simulink model "ALL_JP360_DBW_V6_5_1103"  (R2022a)
settings: Solver=FixedStepAuto  StartTime=0.0  StopTime=inf  FixedStep=0.01  RelTol=1e-3  EnableMultiTasking=on
model workspace (MAT data in the model file):
  g = 9.8
undefined symbols (not defined in the file or in its folder): canChannel, delta_v_p, IPM_Line_C0, IPM_Line_C1, IPM_Line_C2, IPM_Line_C3, M, M_p, MRR_ObjDistX, MRR_ObjDistY, MRR_ObjFusionCamID, MRR_ObjFusionSig, MRR_ObjID, MRR_ObjRelVelX, MRR_ObjRelVelY, MRR_ObjType, MRR_ObjUpdFlg, none, obj_vaild, untracktime, V, videoinput
libraries: canfdmsglib x230, canfdlib x76, slpidlib x24, simulink x18, dspstat3 x14, ctrlSharedLib x1, simulink_extras x1, imaqlib x1, realtime_pacer_lib x1, dspvision x1, visionsinks x1
(part 34 of 55)

== system ALL_JP360_DBW_V6_5_1103/MsgFromCAN/SRR_ADCU_MsgFromCAN/SRR_ADCU_RRR_Freespace_0x1EC ==
  SRR_ADCU_RRR_Freespace_0x1ECFromInData : Inport  OutDataTypeStr=Bus:CAN_FD_MESSAGE_BUS
  Bus Creator : BusCreator  Inputs=104  OutDataTypeStr=Bus:SRR_ADCU_RRR_Freespace_0x1EC  NonVirtualBus=on
  CAN FD Unpack : canfdmsglib/CAN FD Unpack  CANdbFile=V363 SRR Private CAN-V1.3.dbc  MsgList=(none)  MsgName=RRR_Freespace_0x1EC  ProtocolMode=CAN FD  MsgIDType=Standard (11-bit identifier)  MsgIdentifier=492  MsgLength=64  SignalInfo={'RRR_CRCCheck_FSP_MSG2','504','16','BE','unsigned','Standard','0','1','0','0','65535';'RRR_FreespaceSectorConfidence35','12','2','BE','unsigned','Standard','0','1','0','0','3';'RRR_FreespaceSectorConfidence36','30','2','BE','unsigned','Standard','0','1','0','0','3';'RRR_FreespaceSectorConfidence37','32','2','BE','unsigned','Standard','0','1','0','0','3';'RRR_FreespaceSectorConfidence38','50','2','BE','unsigned','Standard','0','1','0','0','3';'RRR_FreespaceSectorConfidence39','68','2','BE','unsigned','Standard','0','1','0','0','3';'RRR_FreespaceSectorConfidence40','86','2','BE','unsigned','Standard','0','1','0','0','3';'RRR_FreespaceSectorConfidence41','88','2','BE','unsigned','Standard','0','1','0','0','3';'RRR_FreespaceSectorConfidence42','106','2','BE','unsigned','Standard','0','1','0','0','3';'RRR_FreespaceSectorConfidence43','124','2','BE','unsigned','Standard','0','1','0','0','3';'RRR_FreespaceSectorConfidence44','142','2','BE','unsigned','Standard','0','1','0','0','3';'RRR_FreespaceSectorConfidence45','144','2','BE','unsigned','Standard','0','1','0','0','3';'RRR_FreespaceSectorConfidence46','162','2','BE','unsigned','Standard','0','1','0','0','3';'RRR_FreespaceSectorConfidence47','180','2','BE','unsigned','Standard','0','1','0','0','3';'RRR_FreespaceSectorConfidence48','198','2','BE','unsigned','Standard','0','1','0','0','3';'RRR_FreespaceSectorConfidence49','200','2','BE','unsigned','Standard','0','1','0','0','3';'RRR_FreespaceSectorConfidence50','218','2','BE','unsigned','Standard','0','1','0','0','3';'RRR_FreespaceSectorConfidence51','236','2','BE','unsigned','Standard','0','1','0','0','3';'RRR_FreespaceSectorConfidence52','254','2','BE','unsigned','Standard','0','1','0','0','3';'RRR_FreespaceSectorConfidence53','256','2','BE','unsigned','Standard','0','1','0','0','3';'RRR_FreespaceSectorConfidence54','274','2','BE','unsigned','Standard','0','1','0','0','3';'RRR_FreespaceSectorConfidence55','292','2','BE','unsigned','Standard','0','1','0','0','3';'RRR_FreespaceSectorConfidence56','310','2','BE','unsigned','Standard','0','1','0','0','3';'RRR_FreespaceSectorConfidence57','312','2','BE','unsigned','Standard','0','1','0','0','3';'RRR_FreespaceSectorConfidence58','330','2','BE','unsigned','Standard','0','1','0','0','3';'RRR_FreespaceSectorConfidence59','348','2','BE','unsigned','Standard','0','1','0','0','3';'RRR_FreespaceSectorConfidence60','366','2','BE','unsigned','Standard','0','1','0','0','3';'RRR_FreespaceSectorConfidence61','368','2','BE','unsigned','Standard','0','1','0','0','3';'RRR_FreespaceSectorConfidence62','386','2','BE','unsigned','Standard','0','1','0','0','3';'RRR_FreespaceSectorConfidence63','404','2','BE','unsigned','Standard','0','1','0','0','3';'RRR_FreespaceSectorConfidence64','422','2','BE','unsigned','Standard','0','1','0','0','3';'RRR_FreespaceSectorConfidence65','424','2','BE','unsigned','Standard','0','1','0','0','3';'RRR_FreespaceSectorConfidence66','442','2','BE','unsigned','Standard','0','1','0','0','3';'RRR_FreespaceSectorConfidence67','460','2','BE','unsigned','Standard','0','1','0','0','3';'RRR_FreespaceSectorConfidence68','478','2','BE','unsigned','Standard','0','1','0','0','3';'RRR_FreespaceSectorDistance35','14','10','BE','unsigned','Standard','0','0.1','0','0','100';'RRR_FreespaceSectorDistance36','16','10','BE','unsigned','Standard','0','0.1','0','0','100';'RRR_FreespaceSectorDistance37','34','10','BE','unsigned','Standard','0','0.1','0','0','100';'RRR_FreespaceSectorDistance38','52','10','BE','unsigned','Standard','0','0.1','0','0','100';'RRR_FreespaceSectorDistance39','70','10','BE','unsigned','Standard','0','0.1','0','0','100';'RRR_FreespaceSectorDistance40','72','10','BE','unsigned','Standard','0','0.1','0','0','100';'RRR_FreespaceSectorDistance41','90','10','BE','unsigned','Standard','0','0.1','0','0','100';'RRR_FreespaceSectorDistance42','108','10','BE','unsigned','Standard','0','0.1','0','0','100';'RRR_FreespaceSectorDistance43','126','10','BE','unsigned','Standard','0','0.1','0','0','100';'RRR_FreespaceSectorDistance44','128','10','BE','unsigned','Standard','0','0.1','0','0','100';'RRR_FreespaceSectorDistance45','146','10','BE','unsigned','Standard','0','0.1','0','0','100';'RRR_FreespaceSectorDistance46','164','10','BE','unsigned','Standard','0','0.1','0','0','100';'RRR_FreespaceSectorDistance47','182','10','BE','unsigned','Standard','0','0.1','0','0','100';'RRR_FreespaceSectorDistance48','184','10','BE','unsigned','Standard','0','0.1','0','0','100';'RRR_FreespaceSectorDistance49','202','10','BE','unsigned','Standard','0','0.1','0','0','100';'RRR_FreespaceSectorDistance50','220','10','BE','unsigned','Standard','0','0.1','0','0','100';'RRR_FreespaceSectorDistance51','238','10','BE','unsigned','Standard','0','0.1','0','0','100';'RRR_FreespaceSectorDistance52','240','10','BE','unsigned','Standard','0','0.1','0','0','100';'RRR_FreespaceSectorDistance53','258','10','BE','unsigned','Standard','0','0.1','0','0','100';'RRR_FreespaceSectorDistance54','276','10','BE','unsigned','Standard','0','0.1','0','0','100';'RRR_FreespaceSectorDistance55','294','10','BE','unsigned','Standard','0','0.1','0','0','100';'RRR_FreespaceSectorDistance56','296','10','BE','unsigned','Standard','0','0.1','0','0','100';'RRR_FreespaceSectorDistance57','314','10','BE','unsigned','Standard','0','0.1','0','0','100';'RRR_FreespaceSectorDistance58','332','10','BE','unsigned','Standard','0','0.1','0','0','100';'RRR_FreespaceSectorDistance59','350','10','BE','unsigned','Standard','0','0.1','0','0','100';'RRR_FreespaceSectorDistance60','352','10','BE','unsigned','Standard','0','0.1','0','0','100';'RRR_FreespaceSectorDistance61','370','10','BE','unsigned','Standard','0','0.1','0','0','100';'RRR_FreespaceSectorDistance62','388','10','BE','unsigned','Standard','0','0.1','0','0','100';'RRR_FreespaceSectorDistance63','406','10','BE','unsigned','Standard','0','0.1','0','0','100';'RRR_FreespaceSectorDistance64','408','10','BE','unsigned','Standard','0','0.1','0','0','100';'RRR_FreespaceSectorDistance65','426','10','BE','unsigned','Standard','0','0.1','0','0','100';'RRR_FreespaceSectorDistance66','444','10','BE','unsigned','Standard','0','0.1','0','0','100';'RRR_FreespaceSectorDistance67','462','10','BE','unsigned','Standard','0','0.1','0','0','100';'RRR_FreespaceSectorDistance68','464','10','BE','unsigned','Standard','0','0.1','0','0','100';'RRR_FreespaceSectorKinestate35','10','2','BE','unsigned','Standard','0','1','0','0','3';'RRR_FreespaceSectorKinestate36','28','2','BE','unsigned','Standard','0','1','0','0','3';'RRR_FreespaceSectorKinestate37','46','2','BE','unsigned','Standard','0','1','0','0','3';'RRR_FreespaceSectorKinestate38','48','2','BE','unsigned','Standard','0','1','0','0','3';'RRR_FreespaceSectorKinestate39','66','2','BE','unsigned','Standard','0','1','0','0','3';'RRR_FreespaceSectorKinestate40','84','2','BE','unsigned','Standard','0','1','0','0','3';'RRR_FreespaceSectorKinestate41','102','2','BE','unsigned','Standard','0','1','0','0','3';'RRR_FreespaceSectorKinestate42','104','2','BE','unsigned','Standard','0','1','0','0','3';'RRR_FreespaceSectorKinestate43','122','2','BE','unsigned','Standard','0','1','0','0','3';'RRR_FreespaceSectorKinestate44','140','2','BE','unsigned','Standard','0','1','0','0','3';'RRR_FreespaceSectorKinestate45','158','2','BE','unsigned','Standard','0','1','0','0','3';'RRR_FreespaceSectorKinestate46','160','2','BE','unsigned','Standard','0','1','0','0','3';'RRR_FreespaceSectorKinestate47','178','2','BE','unsigned','Standard','0','1','0','0','3';'RRR_FreespaceSectorKinestate48','196','2','BE','unsigned','Standard','0','1','0','0','3';'RRR_FreespaceSectorKinestate49','214','2','BE','unsigned','Standard','0','1','0','0','3';'RRR_FreespaceSectorKinestate50','216','2','BE','unsigned','Standard','0','1','0','0','3';'RRR_FreespaceSectorKinestate51','234','2','BE','unsigned','Standard','0','1','0','0','3';'RRR_FreespaceSectorKinestate52','252','2','BE','unsigned','Standard','0','1','0','0','3';'RRR_FreespaceSectorKinestate53','270','2','BE','unsigned','Standard','0','1','0','0','3';'RRR_FreespaceSectorKinestate54','272','2','BE','unsigned','Standard','0','1','0','0','3';'RRR_FreespaceSectorKinestate55','290','2','BE','unsigned','Standard','0','1','0','0','3';'RRR_FreespaceSectorKinestate56','308','2','BE','unsigned','Standard','0','1','0','0','3';'RRR_FreespaceSectorKinestate57','326','2','BE','unsigned','Standard','0','1','0','0','3';'RRR_FreespaceSectorKinestate58','328','2','BE','unsigned','Standard','0','1','0','0','3';'RRR_FreespaceSectorKinestate59','346','2','BE','unsigned','Standard','0','1','0','0','3';'RRR_FreespaceSectorKinestate60','364','2','BE','unsigned','Standard','0','1','0','0','3';'RRR_FreespaceSectorKinestate61','382','2','BE','unsigned','Standard','0','1','0','0','3';'RRR_FreespaceSectorKinestate62','384','2','BE','unsigned','Standard','0','1','0','0','3';'RRR_FreespaceSectorKinestate63','402','2','BE','unsigned','Standard','0','1','0','0','3';'RRR_FreespaceSectorKinestate64','420','2','BE','unsigned','Standard','0','1','0','0','3';'RRR_FreespaceSectorKinestate65','438','2','BE','unsigned','Standard','0','1','0','0','3';'RRR_FreespaceSectorKinestate66','440','2','BE','unsigned','Standard','0','1','0','0','3';'RRR_FreespaceSectorKinestate67','458','2','BE','unsigned','Standard','0','1','0','0','3';'RRR_FreespaceSectorKinestate68','476','2','BE','unsigned','Standard','0','1','0','0','3';'RRR_RollingCounter_FSP_MSG2','488','4','BE','unsigned','Standard','0','1','0','0','15'}  IDPort=off  TimestampPort=off  ErrorPort=off  RemotePort=off  LengthPort=off  StatusPort=off  BRSPort=off  ESIPort=off  DLCPort=off  ApplyMinMax=off
      settings: SourceProductBaseCode=ME,XP,VN  DataFormat=CANdb specified signals
  Data Type Conversion1 : DataTypeConversion  OutDataTypeStr=uint16  SaturateOnIntegerOverflow=off  RndMeth=Floor
  Data Type Conversion{2..35,70..104} (69 alike) : DataTypeConversion  OutDataTypeStr=int8  SaturateOnIntegerOverflow=off  RndMeth=Floor
  Data Type Conversion{36..69} (34 alike) : DataTypeConversion  OutDataTypeStr=single  SaturateOnIntegerOverflow=off  RndMeth=Floor
  SRR_ADCU_RRR_Freespace_0x1ECFromOutData : Outport  OutDataTypeStr=Bus:SRR_ADCU_RRR_Freespace_0x1EC
  wires:
  CAN FD Unpack/1 -> Data Type Conversion1/1
  CAN FD Unpack/2 -> Data Type Conversion2/1
  CAN FD Unpack/3 -> Data Type Conversion3/1
  CAN FD Unpack/4 -> Data Type Conversion4/1
  CAN FD Unpack/5 -> Data Type Conversion5/1
  CAN FD Unpack/6 -> Data Type Conversion6/1
  CAN FD Unpack/7 -> Data Type Conversion7/1
  CAN FD Unpack/8 -> Data Type Conversion8/1
  CAN FD Unpack/9 -> Data Type Conversion9/1
  CAN FD Unpack/10 -> Data Type Conversion10/1
  CAN FD Unpack/11 -> Data Type Conversion11/1
  CAN FD Unpack/12 -> Data Type Conversion12/1
  CAN FD Unpack/13 -> Data Type Conversion13/1
  CAN FD Unpack/14 -> Data Type Conversion14/1
  CAN FD Unpack/15 -> Data Type Conversion15/1
  CAN FD Unpack/16 -> Data Type Conversion16/1
  CAN FD Unpack/17 -> Data Type Conversion17/1
  CAN FD Unpack/18 -> Data Type Conversion18/1
  CAN FD Unpack/19 -> Data Type Conversion19/1
  CAN FD Unpack/20 -> Data Type Conversion20/1
  CAN FD Unpack/21 -> Data Type Conversion21/1
  CAN FD Unpack/22 -> Data Type Conversion22/1
  CAN FD Unpack/23 -> Data Type Conversion23/1
  CAN FD Unpack/24 -> Data Type Conversion24/1
  CAN FD Unpack/25 -> Data Type Conversion25/1
  CAN FD Unpack/26 -> Data Type Conversion26/1
  CAN FD Unpack/27 -> Data Type Conversion27/1
  CAN FD Unpack/28 -> Data Type Conversion28/1
  CAN FD Unpack/29 -> Data Type Conversion29/1
  CAN FD Unpack/30 -> Data Type Conversion30/1
  CAN FD Unpack/31 -> Data Type Conversion31/1
  CAN FD Unpack/32 -> Data Type Conversion32/1
  CAN FD Unpack/33 -> Data Type Conversion33/1
  CAN FD Unpack/34 -> Data Type Conversion34/1
  CAN FD Unpack/35 -> Data Type Conversion35/1
  CAN FD Unpack/36 -> Data Type Conversion36/1
  CAN FD Unpack/37 -> Data Type Conversion37/1
  CAN FD Unpack/38 -> Data Type Conversion38/1
  CAN FD Unpack/39 -> Data Type Conversion39/1
  CAN FD Unpack/40 -> Data Type Conversion40/1
  CAN FD Unpack/41 -> Data Type Conversion41/1
  CAN FD Unpack/42 -> Data Type Conversion42/1
  CAN FD Unpack/43 -> Data Type Conversion43/1
  CAN FD Unpack/44 -> Data Type Conversion44/1
  CAN FD Unpack/45 -> Data Type Conversion45/1
  CAN FD Unpack/46 -> Data Type Conversion46/1
  CAN FD Unpack/47 -> Data Type Conversion47/1
  CAN FD Unpack/48 -> Data Type Conversion48/1
  CAN FD Unpack/49 -> Data Type Conversion49/1
  CAN FD Unpack/50 -> Data Type Conversion50/1
  CAN FD Unpack/51 -> Data Type Conversion51/1
  CAN FD Unpack/52 -> Data Type Conversion52/1
  CAN FD Unpack/53 -> Data Type Conversion53/1
  CAN FD Unpack/54 -> Data Type Conversion54/1
  CAN FD Unpack/55 -> Data Type Conversion55/1
  CAN FD Unpack/56 -> Data Type Conversion56/1
  CAN FD Unpack/57 -> Data Type Conversion57/1
  CAN FD Unpack/58 -> Data Type Conversion58/1
  CAN FD Unpack/59 -> Data Type Conversion59/1
  CAN FD Unpack/60 -> Data Type Conversion60/1
  CAN FD Unpack/61 -> Data Type Conversion61/1
  CAN FD Unpack/62 -> Data Type Conversion62/1
  CAN FD Unpack/63 -> Data Type Conversion63/1
  CAN FD Unpack/64 -> Data Type Conversion64/1
  CAN FD Unpack/65 -> Data Type Conversion65/1
  CAN FD Unpack/66 -> Data Type Conversion66/1
  CAN FD Unpack/67 -> Data Type Conversion67/1
  CAN FD Unpack/68 -> Data Type Conversion68/1
  CAN FD Unpack/69 -> Data Type Conversion69/1
  CAN FD Unpack/70 -> Data Type Conversion70/1
  CAN FD Unpack/71 -> Data Type Conversion71/1
  CAN FD Unpack/72 -> Data Type Conversion72/1
  CAN FD Unpack/73 -> Data Type Conversion73/1
  CAN FD Unpack/74 -> Data Type Conversion74/1
  CAN FD Unpack/75 -> Data Type Conversion75/1
  CAN FD Unpack/76 -> Data Type Conversion76/1
  CAN FD Unpack/77 -> Data Type Conversion77/1
  CAN FD Unpack/78 -> Data Type Conversion78/1
  CAN FD Unpack/79 -> Data Type Conversion79/1
  CAN FD Unpack/80 -> Data Type Conversion80/1
  CAN FD Unpack/81 -> Data Type Conversion81/1
  CAN FD Unpack/82 -> Data Type Conversion82/1
  CAN FD Unpack/83 -> Data Type Conversion83/1
  CAN FD Unpack/84 -> Data Type Conversion84/1
  CAN FD Unpack/85 -> Data Type Conversion85/1
  CAN FD Unpack/86 -> Data Type Conversion86/1
  CAN FD Unpack/87 -> Data Type Conversion87/1
  CAN FD Unpack/88 -> Data Type Conversion88/1
  CAN FD Unpack/89 -> Data Type Conversion89/1
  CAN FD Unpack/90 -> Data Type Conversion90/1
  CAN FD Unpack/91 -> Data Type Conversion91/1
  CAN FD Unpack/92 -> Data Type Conversion92/1
  CAN FD Unpack/93 -> Data Type Conversion93/1
  CAN FD Unpack/94 -> Data Type Conversion94/1
  CAN FD Unpack/95 -> Data Type Conversion95/1
  CAN FD Unpack/96 -> Data Type Conversion96/1
  CAN FD Unpack/97 -> Data Type Conversion97/1
  CAN FD Unpack/98 -> Data Type Conversion98/1
  CAN FD Unpack/99 -> Data Type Conversion99/1
  CAN FD Unpack/100 -> Data Type Conversion100/1
  CAN FD Unpack/101 -> Data Type Conversion101/1
  CAN FD Unpack/102 -> Data Type Conversion102/1
  CAN FD Unpack/103 -> Data Type Conversion103/1
  CAN FD Unpack/104 -> Data Type Conversion104/1
  Data Type Conversion1/1 -> Bus Creator/1  "RRR_CRCCheck_FSP_MSG2"
  Data Type Conversion2/1 -> Bus Creator/2  "RRR_FreespaceSectorConfidence35"
  Data Type Conversion3/1 -> Bus Creator/3  "RRR_FreespaceSectorConfidence36"
  Data Type Conversion4/1 -> Bus Creator/4  "RRR_FreespaceSectorConfidence37"
  Data Type Conversion5/1 -> Bus Creator/5  "RRR_FreespaceSectorConfidence38"
  Data Type Conversion6/1 -> Bus Creator/6  "RRR_FreespaceSectorConfidence39"
  Data Type Conversion7/1 -> Bus Creator/7  "RRR_FreespaceSectorConfidence40"
  Data Type Conversion8/1 -> Bus Creator/8  "RRR_FreespaceSectorConfidence41"
  Data Type Conversion9/1 -> Bus Creator/9  "RRR_FreespaceSectorConfidence42"
  Data Type Conversion10/1 -> Bus Creator/10  "RRR_FreespaceSectorConfidence43"
  Data Type Conversion11/1 -> Bus Creator/11  "RRR_FreespaceSectorConfidence44"
  Data Type Conversion12/1 -> Bus Creator/12  "RRR_FreespaceSectorConfidence45"
  Data Type Conversion13/1 -> Bus Creator/13  "RRR_FreespaceSectorConfidence46"
  Data Type Conversion14/1 -> Bus Creator/14  "RRR_FreespaceSectorConfidence47"
  Data Type Conversion15/1 -> Bus Creator/15  "RRR_FreespaceSectorConfidence48"
  Data Type Conversion16/1 -> Bus Creator/16  "RRR_FreespaceSectorConfidence49"
  Data Type Conversion17/1 -> Bus Creator/17  "RRR_FreespaceSectorConfidence50"
  Data Type Conversion18/1 -> Bus Creator/18  "RRR_FreespaceSectorConfidence51"
  Data Type Conversion19/1 -> Bus Creator/19  "RRR_FreespaceSectorConfidence52"
  Data Type Conversion20/1 -> Bus Creator/20  "RRR_FreespaceSectorConfidence53"
  Data Type Conversion21/1 -> Bus Creator/21  "RRR_FreespaceSectorConfidence54"
  Data Type Conversion22/1 -> Bus Creator/22  "RRR_FreespaceSectorConfidence55"
  Data Type Conversion23/1 -> Bus Creator/23  "RRR_FreespaceSectorConfidence56"
  Data Type Conversion24/1 -> Bus Creator/24  "RRR_FreespaceSectorConfidence57"
  Data Type Conversion25/1 -> Bus Creator/25  "RRR_FreespaceSectorConfidence58"
  Data Type Conversion26/1 -> Bus Creator/26  "RRR_FreespaceSectorConfidence59"
  Data Type Conversion27/1 -> Bus Creator/27  "RRR_FreespaceSectorConfidence60"
  Data Type Conversion28/1 -> Bus Creator/28  "RRR_FreespaceSectorConfidence61"
  Data Type Conversion29/1 -> Bus Creator/29  "RRR_FreespaceSectorConfidence62"
  Data Type Conversion30/1 -> Bus Creator/30  "RRR_FreespaceSectorConfidence63"
  Data Type Conversion31/1 -> Bus Creator/31  "RRR_FreespaceSectorConfidence64"
  Data Type Conversion32/1 -> Bus Creator/32  "RRR_FreespaceSectorConfidence65"
  Data Type Conversion33/1 -> Bus Creator/33  "RRR_FreespaceSectorConfidence66"
  Data Type Conversion34/1 -> Bus Creator/34  "RRR_FreespaceSectorConfidence67"
  Data Type Conversion35/1 -> Bus Creator/35  "RRR_FreespaceSectorConfidence68"
  Data Type Conversion36/1 -> Bus Creator/36  "RRR_FreespaceSectorDistance35"
  Data Type Conversion37/1 -> Bus Creator/37  "RRR_FreespaceSectorDistance36"
  Data Type Conversion38/1 -> Bus Creator/38  "RRR_FreespaceSectorDistance37"
  Data Type Conversion39/1 -> Bus Creator/39  "RRR_FreespaceSectorDistance38"
  Data Type Conversion40/1 -> Bus Creator/40  "RRR_FreespaceSectorDistance39"
  Data Type Conversion41/1 -> Bus Creator/41  "RRR_FreespaceSectorDistance40"
  Data Type Conversion42/1 -> Bus Creator/42  "RRR_FreespaceSectorDistance41"
  Data Type Conversion43/1 -> Bus Creator/43  "RRR_FreespaceSectorDistance42"
  Data Type Conversion44/1 -> Bus Creator/44  "RRR_FreespaceSectorDistance43"
  Data Type Conversion45/1 -> Bus Creator/45  "RRR_FreespaceSectorDistance44"
  Data Type Conversion46/1 -> Bus Creator/46  "RRR_FreespaceSectorDistance45"
  Data Type Conversion47/1 -> Bus Creator/47  "RRR_FreespaceSectorDistance46"
  Data Type Conversion48/1 -> Bus Creator/48  "RRR_FreespaceSectorDistance47"
  Data Type Conversion49/1 -> Bus Creator/49  "RRR_FreespaceSectorDistance48"
  Data Type Conversion50/1 -> Bus Creator/50  "RRR_FreespaceSectorDistance49"
  Data Type Conversion51/1 -> Bus Creator/51  "RRR_FreespaceSectorDistance50"
  Data Type Conversion52/1 -> Bus Creator/52  "RRR_FreespaceSectorDistance51"
  Data Type Conversion53/1 -> Bus Creator/53  "RRR_FreespaceSectorDistance52"
  Data Type Conversion54/1 -> Bus Creator/54  "RRR_FreespaceSectorDistance53"
  Data Type Conversion55/1 -> Bus Creator/55  "RRR_FreespaceSectorDistance54"
  Data Type Conversion56/1 -> Bus Creator/56  "RRR_FreespaceSectorDistance55"
  Data Type Conversion57/1 -> Bus Creator/57  "RRR_FreespaceSectorDistance56"
  Data Type Conversion58/1 -> Bus Creator/58  "RRR_FreespaceSectorDistance57"
  Data Type Conversion59/1 -> Bus Creator/59  "RRR_FreespaceSectorDistance58"
  Data Type Conversion60/1 -> Bus Creator/60  "RRR_FreespaceSectorDistance59"
  Data Type Conversion61/1 -> Bus Creator/61  "RRR_FreespaceSectorDistance60"
  Data Type Conversion62/1 -> Bus Creator/62  "RRR_FreespaceSectorDistance61"
  Data Type Conversion63/1 -> Bus Creator/63  "RRR_FreespaceSectorDistance62"
  Data Type Conversion64/1 -> Bus Creator/64  "RRR_FreespaceSectorDistance63"
  Data Type Conversion65/1 -> Bus Creator/65  "RRR_FreespaceSectorDistance64"
  Data Type Conversion66/1 -> Bus Creator/66  "RRR_FreespaceSectorDistance65"
  Data Type Conversion67/1 -> Bus Creator/67  "RRR_FreespaceSectorDistance66"
  Data Type Conversion68/1 -> Bus Creator/68  "RRR_FreespaceSectorDistance67"
  Data Type Conversion69/1 -> Bus Creator/69  "RRR_FreespaceSectorDistance68"
  Data Type Conversion70/1 -> Bus Creator/70  "RRR_FreespaceSectorKinestate35"
  Data Type Conversion71/1 -> Bus Creator/71  "RRR_FreespaceSectorKinestate36"
  Data Type Conversion72/1 -> Bus Creator/72  "RRR_FreespaceSectorKinestate37"
  Data Type Conversion73/1 -> Bus Creator/73  "RRR_FreespaceSectorKinestate38"
  Data Type Conversion74/1 -> Bus Creator/74  "RRR_FreespaceSectorKinestate39"
  Data Type Conversion75/1 -> Bus Creator/75  "RRR_FreespaceSectorKinestate40"
  Data Type Conversion76/1 -> Bus Creator/76  "RRR_FreespaceSectorKinestate41"
  Data Type Conversion77/1 -> Bus Creator/77  "RRR_FreespaceSectorKinestate42"
  Data Type Conversion78/1 -> Bus Creator/78  "RRR_FreespaceSectorKinestate43"
  Data Type Conversion79/1 -> Bus Creator/79  "RRR_FreespaceSectorKinestate44"
  Data Type Conversion80/1 -> Bus Creator/80  "RRR_FreespaceSectorKinestate45"
  Data Type Conversion81/1 -> Bus Creator/81  "RRR_FreespaceSectorKinestate46"
  Data Type Conversion82/1 -> Bus Creator/82  "RRR_FreespaceSectorKinestate47"
  Data Type Conversion83/1 -> Bus Creator/83  "RRR_FreespaceSectorKinestate48"
  Data Type Conversion84/1 -> Bus Creator/84  "RRR_FreespaceSectorKinestate49"
  Data Type Conversion85/1 -> Bus Creator/85  "RRR_FreespaceSectorKinestate50"
  Data Type Conversion86/1 -> Bus Creator/86  "RRR_FreespaceSectorKinestate51"
  Data Type Conversion87/1 -> Bus Creator/87  "RRR_FreespaceSectorKinestate52"
  Data Type Conversion88/1 -> Bus Creator/88  "RRR_FreespaceSectorKinestate53"
  Data Type Conversion89/1 -> Bus Creator/89  "RRR_FreespaceSectorKinestate54"
  Data Type Conversion90/1 -> Bus Creator/90  "RRR_FreespaceSectorKinestate55"
  Data Type Conversion91/1 -> Bus Creator/91  "RRR_FreespaceSectorKinestate56"
  Data Type Conversion92/1 -> Bus Creator/92  "RRR_FreespaceSectorKinestate57"
  Data Type Conversion93/1 -> Bus Creator/93  "RRR_FreespaceSectorKinestate58"
  Data Type Conversion94/1 -> Bus Creator/94  "RRR_FreespaceSectorKinestate59"
  Data Type Conversion95/1 -> Bus Creator/95  "RRR_FreespaceSectorKinestate60"
  Data Type Conversion96/1 -> Bus Creator/96  "RRR_FreespaceSectorKinestate61"
  Data Type Conversion97/1 -> Bus Creator/97  "RRR_FreespaceSectorKinestate62"
  Data Type Conversion98/1 -> Bus Creator/98  "RRR_FreespaceSectorKinestate63"
  Data Type Conversion99/1 -> Bus Creator/99  "RRR_FreespaceSectorKinestate64"
  Data Type Conversion100/1 -> Bus Creator/100  "RRR_FreespaceSectorKinestate65"
  Data Type Conversion101/1 -> Bus Creator/101  "RRR_FreespaceSectorKinestate66"
  Data Type Conversion102/1 -> Bus Creator/102  "RRR_FreespaceSectorKinestate67"
  Data Type Conversion103/1 -> Bus Creator/103  "RRR_FreespaceSectorKinestate68"
  Data Type Conversion104/1 -> Bus Creator/104  "RRR_RollingCounter_FSP_MSG2"
  Bus Creator/1 -> SRR_ADCU_RRR_Freespace_0x1ECFromOutData/1  "SRR_ADCU_RRR_Freespace_0x1ECFromOutData"
  SRR_ADCU_RRR_Freespace_0x1ECFromInData/1 -> CAN FD Unpack/1  "SRR_ADCU_RRR_Freespace_0x1ECFromInData"

== system ALL_JP360_DBW_V6_5_1103/MsgFromCAN/SRR_ADCU_MsgFromCAN/SRR_ADCU_RRR_Freespace_0x1ED ==
  SRR_ADCU_RRR_Freespace_0x1EDFromInData : Inport  OutDataTypeStr=Bus:CAN_FD_MESSAGE_BUS
  Bus Creator : BusCreator  Inputs=104  OutDataTypeStr=Bus:SRR_ADCU_RRR_Freespace_0x1ED  NonVirtualBus=on
  CAN FD Unpack : canfdmsglib/CAN FD Unpack  CANdbFile=V363 SRR Private CAN-V1.3.dbc  MsgList=(none)  MsgName=RRR_Freespace_0x1ED  ProtocolMode=CAN FD  MsgIDType=Standard (11-bit identifier)  MsgIdentifier=493  MsgLength=64  SignalInfo={'RRR_CRCCheck_FSP_MSG3','504','16','BE','unsigned','Standard','0','1','0','0','65535';'RRR_FreespaceSectorConfidence100','442','2','BE','unsigned','Standard','0','1','0','0','3';'RRR_FreespaceSectorConfidence101','460','2','BE','unsigned','Standard','0','1','0','0','3';'RRR_FreespaceSectorConfidence102','478','2','BE','unsigned','Standard','0','1','0','0','3';'RRR_FreespaceSectorConfidence69','12','2','BE','unsigned','Standard','0','1','0','0','3';'RRR_FreespaceSectorConfidence70','30','2','BE','unsigned','Standard','0','1','0','0','3';'RRR_FreespaceSectorConfidence71','32','2','BE','unsigned','Standard','0','1','0','0','3';'RRR_FreespaceSectorConfidence72','50','2','BE','unsigned','Standard','0','1','0','0','3';'RRR_FreespaceSectorConfidence73','68','2','BE','unsigned','Standard','0','1','0','0','3';'RRR_FreespaceSectorConfidence74','86','2','BE','unsigned','Standard','0','1','0','0','3';'RRR_FreespaceSectorConfidence75','88','2','BE','unsigned','Standard','0','1','0','0','3';'RRR_FreespaceSectorConfidence76','106','2','BE','unsigned','Standard','0','1','0','0','3';'RRR_FreespaceSectorConfidence77','124','2','BE','unsigned','Standard','0','1','0','0','3';'RRR_FreespaceSectorConfidence78','142','2','BE','unsigned','Standard','0','1','0','0','3';'RRR_FreespaceSectorConfidence79','144','2','BE','unsigned','Standard','0','1','0','0','3';'RRR_FreespaceSectorConfidence80','162','2','BE','unsigned','Standard','0','1','0','0','3';'RRR_FreespaceSectorConfidence81','180','2','BE','unsigned','Standard','0','1','0','0','3';'RRR_FreespaceSectorConfidence82','198','2','BE','unsigned','Standard','0','1','0','0','3';'RRR_FreespaceSectorConfidence83','200','2','BE','unsigned','Standard','0','1','0','0','3';'RRR_FreespaceSectorConfidence84','218','2','BE','unsigned','Standard','0','1','0','0','3';'RRR_FreespaceSectorConfidence85','236','2','BE','unsigned','Standard','0','1','0','0','3';'RRR_FreespaceSectorConfidence86','254','2','BE','unsigned','Standard','0','1','0','0','3';'RRR_FreespaceSectorConfidence87','256','2','BE','unsigned','Standard','0','1','0','0','3';'RRR_FreespaceSectorConfidence88','274','2','BE','unsigned','Standard','0','1','0','0','3';'RRR_FreespaceSectorConfidence89','292','2','BE','unsigned','Standard','0','1','0','0','3';'RRR_FreespaceSectorConfidence90','310','2','BE','unsigned','Standard','0','1','0','0','3';'RRR_FreespaceSectorConfidence91','312','2','BE','unsigned','Standard','0','1','0','0','3';'RRR_FreespaceSectorConfidence92','330','2','BE','unsigned','Standard','0','1','0','0','3';'RRR_FreespaceSectorConfidence93','348','2','BE','unsigned','Standard','0','1','0','0','3';'RRR_FreespaceSectorConfidence94','366','2','BE','unsigned','Standard','0','1','0','0','3';'RRR_FreespaceSectorConfidence95','368','2','BE','unsigned','Standard','0','1','0','0','3';'RRR_FreespaceSectorConfidence96','386','2','BE','unsigned','Standard','0','1','0','0','3';'RRR_FreespaceSectorConfidence97','404','2','BE','unsigned','Standard','0','1','0','0','3';'RRR_FreespaceSectorConfidence98','422','2','BE','unsigned','Standard','0','1','0','0','3';'RRR_FreespaceSectorConfidence99','424','2','BE','unsigned','Standard','0','1','0','0','3';'RRR_FreespaceSectorDistance100','444','10','BE','unsigned','Standard','0','0.1','0','0','100';'RRR_FreespaceSectorDistance101','462','10','BE','unsigned','Standard','0','0.1','0','0','100';'RRR_FreespaceSectorDistance102','464','10','BE','unsigned','Standard','0','0.1','0','0','100';'RRR_FreespaceSectorDistance69','14','10','BE','unsigned','Standard','0','0.1','0','0','100';'RRR_FreespaceSectorDistance70','16','10','BE','unsigned','Standard','0','0.1','0','0','100';'RRR_FreespaceSectorDistance71','34','10','BE','unsigned','Standard','0','0.1','0','0','100';'RRR_FreespaceSectorDistance72','52','10','BE','unsigned','Standard','0','0.1','0','0','100';'RRR_FreespaceSectorDistance73','70','10','BE','unsigned','Standard','0','0.1','0','0','100';'RRR_FreespaceSectorDistance74','72','10','BE','unsigned','Standard','0','0.1','0','0','100';'RRR_FreespaceSectorDistance75','90','10','BE','unsigned','Standard','0','0.1','0','0','100';'RRR_FreespaceSectorDistance76','108','10','BE','unsigned','Standard','0','0.1','0','0','100';'RRR_FreespaceSectorDistance77','126','10','BE','unsigned','Standard','0','0.1','0','0','100';'RRR_FreespaceSectorDistance78','128','10','BE','unsigned','Standard','0','0.1','0','0','100';'RRR_FreespaceSectorDistance79','146','10','BE','unsigned','Standard','0','0.1','0','0','100';'RRR_FreespaceSectorDistance80','164','10','BE','unsigned','Standard','0','0.1','0','0','100';'RRR_FreespaceSectorDistance81','182','10','BE','unsigned','Standard','0','0.1','0','0','100';'RRR_FreespaceSectorDistance82','184','10','BE','unsigned','Standard','0','0.1','0','0','100';'RRR_FreespaceSectorDistance83','202','10','BE','unsigned','Standard','0','0.1','0','0','100';'RRR_FreespaceSectorDistance84','220','10','BE','unsigned','Standard','0','0.1','0','0','100';'RRR_FreespaceSectorDistance85','238','10','BE','unsigned','Standard','0','0.1','0','0','100';'RRR_FreespaceSectorDistance86','240','10','BE','unsigned','Standard','0','0.1','0','0','100';'RRR_FreespaceSectorDistance87','258','10','BE','unsigned','Standard','0','0.1','0','0','100';'RRR_FreespaceSectorDistance88','276','10','BE','unsigned','Standard','0','0.1','0','0','100';'RRR_FreespaceSectorDistance89','294','10','BE','unsigned','Standard','0','0.1','0','0','100';'RRR_FreespaceSectorDistance90','296','10','BE','unsigned','Standard','0','0.1','0','0','100';'RRR_FreespaceSectorDistance91','314','10','BE','unsigned','Standard','0','0.1','0','0','100';'RRR_FreespaceSectorDistance92','332','10','BE','unsigned','Standard','0','0.1','0','0','100';'RRR_FreespaceSectorDistance93','350','10','BE','unsigned','Standard','0','0.1','0','0','100';'RRR_FreespaceSectorDistance94','352','10','BE','unsigned','Standard','0','0.1','0','0','100';'RRR_FreespaceSectorDistance95','370','10','BE','unsigned','Standard','0','0.1','0','0','100';'RRR_FreespaceSectorDistance96','388','10','BE','unsigned','Standard','0','0.1','0','0','100';'RRR_FreespaceSectorDistance97','406','10','BE','unsigned','Standard','0','0.1','0','0','100';'RRR_FreespaceSectorDistance98','408','10','BE','unsigned','Standard','0','0.1','0','0','100';'RRR_FreespaceSectorDistance99','426','10','BE','unsigned','Standard','0','0.1','0','0','100';'RRR_FreespaceSectorKinestate100','440','2','BE','unsigned','Standard','0','1','0','0','3';'RRR_FreespaceSectorKinestate101','458','2','BE','unsigned','Standard','0','1','0','0','3';'RRR_FreespaceSectorKinestate102','476','2','BE','unsigned','Standard','0','1','0','0','3';'RRR_FreespaceSectorKinestate69','10','2','BE','unsigned','Standard','0','1','0','0','3';'RRR_FreespaceSectorKinestate70','28','2','BE','unsigned','Standard','0','1','0','0','3';'RRR_FreespaceSectorKinestate71','46','2','BE','unsigned','Standard','0','1','0','0','3';'RRR_FreespaceSectorKinestate72','48','2','BE','unsigned','Standard','0','1','0','0','3';'RRR_FreespaceSectorKinestate73','66','2','BE','unsigned','Standard','0','1','0','0','3';'RRR_FreespaceSectorKinestate74','84','2','BE','unsigned','Standard','0','1','0','0','3';'RRR_FreespaceSectorKinestate75','102','2','BE','unsigned','Standard','0','1','0','0','3';'RRR_FreespaceSectorKinestate76','104','2','BE','unsigned','Standard','0','1','0','0','3';'RRR_FreespaceSectorKinestate77','122','2','BE','unsigned','Standard','0','1','0','0','3';'RRR_FreespaceSectorKinestate78','140','2','BE','unsigned','Standard','0','1','0','0','3';'RRR_FreespaceSectorKinestate79','158','2','BE','unsigned','Standard','0','1','0','0','3';'RRR_FreespaceSectorKinestate80','160','2','BE','unsigned','Standard','0','1','0','0','3';'RRR_FreespaceSectorKinestate81','178','2','BE','unsigned','Standard','0','1','0','0','3';'RRR_FreespaceSectorKinestate82','196','2','BE','unsigned','Standard','0','1','0','0','3';'RRR_FreespaceSectorKinestate83','214','2','BE','unsigned','Standard','0','1','0','0','3';'RRR_FreespaceSectorKinestate84','216','2','BE','unsigned','Standard','0','1','0','0','3';'RRR_FreespaceSectorKinestate85','234','2','BE','unsigned','Standard','0','1','0','0','3';'RRR_FreespaceSectorKinestate86','252','2','BE','unsigned','Standard','0','1','0','0','3';'RRR_FreespaceSectorKinestate87','270','2','BE','unsigned','Standard','0','1','0','0','3';'RRR_FreespaceSectorKinestate88','272','2','BE','unsigned','Standard','0','1','0','0','3';'RRR_FreespaceSectorKinestate89','290','2','BE','unsigned','Standard','0','1','0','0','3';'RRR_FreespaceSectorKinestate90','308','2','BE','unsigned','Standard','0','1','0','0','3';'RRR_FreespaceSectorKinestate91','326','2','BE','unsigned','Standard','0','1','0','0','3';'RRR_FreespaceSectorKinestate92','328','2','BE','unsigned','Standard','0','1','0','0','3';'RRR_FreespaceSectorKinestate93','346','2','BE','unsigned','Standard','0','1','0','0','3';'RRR_FreespaceSectorKinestate94','364','2','BE','unsigned','Standard','0','1','0','0','3';'RRR_FreespaceSectorKinestate95','382','2','BE','unsigned','Standard','0','1','0','0','3';'RRR_FreespaceSectorKinestate96','384','2','BE','unsigned','Standard','0','1','0','0','3';'RRR_FreespaceSectorKinestate97','402','2','BE','unsigned','Standard','0','1','0','0','3';'RRR_FreespaceSectorKinestate98','420','2','BE','unsigned','Standard','0','1','0','0','3';'RRR_FreespaceSectorKinestate99','438','2','BE','unsigned','Standard','0','1','0','0','3';'RRR_RollingCounter_FSP_MSG3','488','4','BE','unsigned','Standard','0','1','0','0','15'}  IDPort=off  TimestampPort=off  ErrorPort=off  RemotePort=off  LengthPort=off  StatusPort=off  BRSPort=off  ESIPort=off  DLCPort=off  ApplyMinMax=off
      settings: SourceProductBaseCode=ME,XP,VN  DataFormat=CANdb specified signals
  Data Type Conversion1 : DataTypeConversion  OutDataTypeStr=uint16  SaturateOnIntegerOverflow=off  RndMeth=Floor
  Data Type Conversion{2..35,70..104} (69 alike) : DataTypeConversion  OutDataTypeStr=int8  SaturateOnIntegerOverflow=off  RndMeth=Floor
  Data Type Conversion{36..69} (34 alike) : DataTypeConversion  OutDataTypeStr=single  SaturateOnIntegerOverflow=off  RndMeth=Floor
  SRR_ADCU_RRR_Freespace_0x1EDFromOutData : Outport  OutDataTypeStr=Bus:SRR_ADCU_RRR_Freespace_0x1ED
  wires:
  CAN FD Unpack/1 -> Data Type Conversion1/1
  CAN FD Unpack/2 -> Data Type Conversion2/1
  CAN FD Unpack/3 -> Data Type Conversion3/1
  CAN FD Unpack/4 -> Data Type Conversion4/1
  CAN FD Unpack/5 -> Data Type Conversion5/1
  CAN FD Unpack/6 -> Data Type Conversion6/1
  CAN FD Unpack/7 -> Data Type Conversion7/1
  CAN FD Unpack/8 -> Data Type Conversion8/1
  CAN FD Unpack/9 -> Data Type Conversion9/1
  CAN FD Unpack/10 -> Data Type Conversion10/1
  CAN FD Unpack/11 -> Data Type Conversion11/1
  CAN FD Unpack/12 -> Data Type Conversion12/1
  CAN FD Unpack/13 -> Data Type Conversion13/1
  CAN FD Unpack/14 -> Data Type Conversion14/1
  CAN FD Unpack/15 -> Data Type Conversion15/1
  CAN FD Unpack/16 -> Data Type Conversion16/1
  CAN FD Unpack/17 -> Data Type Conversion17/1
  CAN FD Unpack/18 -> Data Type Conversion18/1
  CAN FD Unpack/19 -> Data Type Conversion19/1
  CAN FD Unpack/20 -> Data Type Conversion20/1
  CAN FD Unpack/21 -> Data Type Conversion21/1
  CAN FD Unpack/22 -> Data Type Conversion22/1
  CAN FD Unpack/23 -> Data Type Conversion23/1
  CAN FD Unpack/24 -> Data Type Conversion24/1
  CAN FD Unpack/25 -> Data Type Conversion25/1
  CAN FD Unpack/26 -> Data Type Conversion26/1
  CAN FD Unpack/27 -> Data Type Conversion27/1
  CAN FD Unpack/28 -> Data Type Conversion28/1
  CAN FD Unpack/29 -> Data Type Conversion29/1
  CAN FD Unpack/30 -> Data Type Conversion30/1
  CAN FD Unpack/31 -> Data Type Conversion31/1
  CAN FD Unpack/32 -> Data Type Conversion32/1
  CAN FD Unpack/33 -> Data Type Conversion33/1
  CAN FD Unpack/34 -> Data Type Conversion34/1
  CAN FD Unpack/35 -> Data Type Conversion35/1
  CAN FD Unpack/36 -> Data Type Conversion36/1
  CAN FD Unpack/37 -> Data Type Conversion37/1
  CAN FD Unpack/38 -> Data Type Conversion38/1
  CAN FD Unpack/39 -> Data Type Conversion39/1
  CAN FD Unpack/40 -> Data Type Conversion40/1
  CAN FD Unpack/41 -> Data Type Conversion41/1
  CAN FD Unpack/42 -> Data Type Conversion42/1
  CAN FD Unpack/43 -> Data Type Conversion43/1
  CAN FD Unpack/44 -> Data Type Conversion44/1
  CAN FD Unpack/45 -> Data Type Conversion45/1
  CAN FD Unpack/46 -> Data Type Conversion46/1
  CAN FD Unpack/47 -> Data Type Conversion47/1
  CAN FD Unpack/48 -> Data Type Conversion48/1
  CAN FD Unpack/49 -> Data Type Conversion49/1
  CAN FD Unpack/50 -> Data Type Conversion50/1
  CAN FD Unpack/51 -> Data Type Conversion51/1
  CAN FD Unpack/52 -> Data Type Conversion52/1
  CAN FD Unpack/53 -> Data Type Conversion53/1
  CAN FD Unpack/54 -> Data Type Conversion54/1
  CAN FD Unpack/55 -> Data Type Conversion55/1
  CAN FD Unpack/56 -> Data Type Conversion56/1
  CAN FD Unpack/57 -> Data Type Conversion57/1
  CAN FD Unpack/58 -> Data Type Conversion58/1
  CAN FD Unpack/59 -> Data Type Conversion59/1
  CAN FD Unpack/60 -> Data Type Conversion60/1
  CAN FD Unpack/61 -> Data Type Conversion61/1
  CAN FD Unpack/62 -> Data Type Conversion62/1
  CAN FD Unpack/63 -> Data Type Conversion63/1
  CAN FD Unpack/64 -> Data Type Conversion64/1
  CAN FD Unpack/65 -> Data Type Conversion65/1
  CAN FD Unpack/66 -> Data Type Conversion66/1
  CAN FD Unpack/67 -> Data Type Conversion67/1
  CAN FD Unpack/68 -> Data Type Conversion68/1
  CAN FD Unpack/69 -> Data Type Conversion69/1
  CAN FD Unpack/70 -> Data Type Conversion70/1
  CAN FD Unpack/71 -> Data Type Conversion71/1
  CAN FD Unpack/72 -> Data Type Conversion72/1
  CAN FD Unpack/73 -> Data Type Conversion73/1
  CAN FD Unpack/74 -> Data Type Conversion74/1
  CAN FD Unpack/75 -> Data Type Conversion75/1
  CAN FD Unpack/76 -> Data Type Conversion76/1
  CAN FD Unpack/77 -> Data Type Conversion77/1
  CAN FD Unpack/78 -> Data Type Conversion78/1
  CAN FD Unpack/79 -> Data Type Conversion79/1
  CAN FD Unpack/80 -> Data Type Conversion80/1
  CAN FD Unpack/81 -> Data Type Conversion81/1
  CAN FD Unpack/82 -> Data Type Conversion82/1
  CAN FD Unpack/83 -> Data Type Conversion83/1
  CAN FD Unpack/84 -> Data Type Conversion84/1
  CAN FD Unpack/85 -> Data Type Conversion85/1
  CAN FD Unpack/86 -> Data Type Conversion86/1
  CAN FD Unpack/87 -> Data Type Conversion87/1
  CAN FD Unpack/88 -> Data Type Conversion88/1
  CAN FD Unpack/89 -> Data Type Conversion89/1
  CAN FD Unpack/90 -> Data Type Conversion90/1
  CAN FD Unpack/91 -> Data Type Conversion91/1
  CAN FD Unpack/92 -> Data Type Conversion92/1
  CAN FD Unpack/93 -> Data Type Conversion93/1
  CAN FD Unpack/94 -> Data Type Conversion94/1
  CAN FD Unpack/95 -> Data Type Conversion95/1
  CAN FD Unpack/96 -> Data Type Conversion96/1
  CAN FD Unpack/97 -> Data Type Conversion97/1
  CAN FD Unpack/98 -> Data Type Conversion98/1
  CAN FD Unpack/99 -> Data Type Conversion99/1
  CAN FD Unpack/100 -> Data Type Conversion100/1
  CAN FD Unpack/101 -> Data Type Conversion101/1
  CAN FD Unpack/102 -> Data Type Conversion102/1
  CAN FD Unpack/103 -> Data Type Conversion103/1
  CAN FD Unpack/104 -> Data Type Conversion104/1
  Data Type Conversion1/1 -> Bus Creator/1  "RRR_CRCCheck_FSP_MSG3"
  Data Type Conversion2/1 -> Bus Creator/2  "RRR_FreespaceSectorConfidence100"
  Data Type Conversion3/1 -> Bus Creator/3  "RRR_FreespaceSectorConfidence101"
  Data Type Conversion4/1 -> Bus Creator/4  "RRR_FreespaceSectorConfidence102"
  Data Type Conversion5/1 -> Bus Creator/5  "RRR_FreespaceSectorConfidence69"
  Data Type Conversion6/1 -> Bus Creator/6  "RRR_FreespaceSectorConfidence70"
  Data Type Conversion7/1 -> Bus Creator/7  "RRR_FreespaceSectorConfidence71"
  Data Type Conversion8/1 -> Bus Creator/8  "RRR_FreespaceSectorConfidence72"
  Data Type Conversion9/1 -> Bus Creator/9  "RRR_FreespaceSectorConfidence73"
  Data Type Conversion10/1 -> Bus Creator/10  "RRR_FreespaceSectorConfidence74"
  Data Type Conversion11/1 -> Bus Creator/11  "RRR_FreespaceSectorConfidence75"
  Data Type Conversion12/1 -> Bus Creator/12  "RRR_FreespaceSectorConfidence76"
  Data Type Conversion13/1 -> Bus Creator/13  "RRR_FreespaceSectorConfidence77"
  Data Type Conversion14/1 -> Bus Creator/14  "RRR_FreespaceSectorConfidence78"
  Data Type Conversion15/1 -> Bus Creator/15  "RRR_FreespaceSectorConfidence79"
  Data Type Conversion16/1 -> Bus Creator/16  "RRR_FreespaceSectorConfidence80"
  Data Type Conversion17/1 -> Bus Creator/17  "RRR_FreespaceSectorConfidence81"
  Data Type Conversion18/1 -> Bus Creator/18  "RRR_FreespaceSectorConfidence82"
  Data Type Conversion19/1 -> Bus Creator/19  "RRR_FreespaceSectorConfidence83"
  Data Type Conversion20/1 -> Bus Creator/20  "RRR_FreespaceSectorConfidence84"
  Data Type Conversion21/1 -> Bus Creator/21  "RRR_FreespaceSectorConfidence85"
  Data Type Conversion22/1 -> Bus Creator/22  "RRR_FreespaceSectorConfidence86"
  Data Type Conversion23/1 -> Bus Creator/23  "RRR_FreespaceSectorConfidence87"
  Data Type Conversion24/1 -> Bus Creator/24  "RRR_FreespaceSectorConfidence88"
  Data Type Conversion25/1 -> Bus Creator/25  "RRR_FreespaceSectorConfidence89"
  Data Type Conversion26/1 -> Bus Creator/26  "RRR_FreespaceSectorConfidence90"
  Data Type Conversion27/1 -> Bus Creator/27  "RRR_FreespaceSectorConfidence91"
  Data Type Conversion28/1 -> Bus Creator/28  "RRR_FreespaceSectorConfidence92"
  Data Type Conversion29/1 -> Bus Creator/29  "RRR_FreespaceSectorConfidence93"
  Data Type Conversion30/1 -> Bus Creator/30  "RRR_FreespaceSectorConfidence94"
  Data Type Conversion31/1 -> Bus Creator/31  "RRR_FreespaceSectorConfidence95"
  Data Type Conversion32/1 -> Bus Creator/32  "RRR_FreespaceSectorConfidence96"
  Data Type Conversion33/1 -> Bus Creator/33  "RRR_FreespaceSectorConfidence97"
  Data Type Conversion34/1 -> Bus Creator/34  "RRR_FreespaceSectorConfidence98"
  Data Type Conversion35/1 -> Bus Creator/35  "RRR_FreespaceSectorConfidence99"
  Data Type Conversion36/1 -> Bus Creator/36  "RRR_FreespaceSectorDistance100"
  Data Type Conversion37/1 -> Bus Creator/37  "RRR_FreespaceSectorDistance101"
  Data Type Conversion38/1 -> Bus Creator/38  "RRR_FreespaceSectorDistance102"
  Data Type Conversion39/1 -> Bus Creator/39  "RRR_FreespaceSectorDistance69"
  Data Type Conversion40/1 -> Bus Creator/40  "RRR_FreespaceSectorDistance70"
  Data Type Conversion41/1 -> Bus Creator/41  "RRR_FreespaceSectorDistance71"
  Data Type Conversion42/1 -> Bus Creator/42  "RRR_FreespaceSectorDistance72"
  Data Type Conversion43/1 -> Bus Creator/43  "RRR_FreespaceSectorDistance73"
  Data Type Conversion44/1 -> Bus Creator/44  "RRR_FreespaceSectorDistance74"
  Data Type Conversion45/1 -> Bus Creator/45  "RRR_FreespaceSectorDistance75"
  Data Type Conversion46/1 -> Bus Creator/46  "RRR_FreespaceSectorDistance76"
  Data Type Conversion47/1 -> Bus Creator/47  "RRR_FreespaceSectorDistance77"
  Data Type Conversion48/1 -> Bus Creator/48  "RRR_FreespaceSectorDistance78"
  Data Type Conversion49/1 -> Bus Creator/49  "RRR_FreespaceSectorDistance79"
  Data Type Conversion50/1 -> Bus Creator/50  "RRR_FreespaceSectorDistance80"
  Data Type Conversion51/1 -> Bus Creator/51  "RRR_FreespaceSectorDistance81"
  Data Type Conversion52/1 -> Bus Creator/52  "RRR_FreespaceSectorDistance82"
  Data Type Conversion53/1 -> Bus Creator/53  "RRR_FreespaceSectorDistance83"
  Data Type Conversion54/1 -> Bus Creator/54  "RRR_FreespaceSectorDistance84"
  Data Type Conversion55/1 -> Bus Creator/55  "RRR_FreespaceSectorDistance85"
  Data Type Conversion56/1 -> Bus Creator/56  "RRR_FreespaceSectorDistance86"
  Data Type Conversion57/1 -> Bus Creator/57  "RRR_FreespaceSectorDistance87"
  Data Type Conversion58/1 -> Bus Creator/58  "RRR_FreespaceSectorDistance88"
  Data Type Conversion59/1 -> Bus Creator/59  "RRR_FreespaceSectorDistance89"
  Data Type Conversion60/1 -> Bus Creator/60  "RRR_FreespaceSectorDistance90"
  Data Type Conversion61/1 -> Bus Creator/61  "RRR_FreespaceSectorDistance91"
  Data Type Conversion62/1 -> Bus Creator/62  "RRR_FreespaceSectorDistance92"
  Data Type Conversion63/1 -> Bus Creator/63  "RRR_FreespaceSectorDistance93"
  Data Type Conversion64/1 -> Bus Creator/64  "RRR_FreespaceSectorDistance94"
  Data Type Conversion65/1 -> Bus Creator/65  "RRR_FreespaceSectorDistance95"
  Data Type Conversion66/1 -> Bus Creator/66  "RRR_FreespaceSectorDistance96"
  Data Type Conversion67/1 -> Bus Creator/67  "RRR_FreespaceSectorDistance97"
  Data Type Conversion68/1 -> Bus Creator/68  "RRR_FreespaceSectorDistance98"
  Data Type Conversion69/1 -> Bus Creator/69  "RRR_FreespaceSectorDistance99"
  Data Type Conversion70/1 -> Bus Creator/70  "RRR_FreespaceSectorKinestate100"
  Data Type Conversion71/1 -> Bus Creator/71  "RRR_FreespaceSectorKinestate101"
  Data Type Conversion72/1 -> Bus Creator/72  "RRR_FreespaceSectorKinestate102"
  Data Type Conversion73/1 -> Bus Creator/73  "RRR_FreespaceSectorKinestate69"
  Data Type Conversion74/1 -> Bus Creator/74  "RRR_FreespaceSectorKinestate70"
  Data Type Conversion75/1 -> Bus Creator/75  "RRR_FreespaceSectorKinestate71"
  Data Type Conversion76/1 -> Bus Creator/76  "RRR_FreespaceSectorKinestate72"
  Data Type Conversion77/1 -> Bus Creator/77  "RRR_FreespaceSectorKinestate73"
  Data Type Conversion78/1 -> Bus Creator/78  "RRR_FreespaceSectorKinestate74"
  Data Type Conversion79/1 -> Bus Creator/79  "RRR_FreespaceSectorKinestate75"
  Data Type Conversion80/1 -> Bus Creator/80  "RRR_FreespaceSectorKinestate76"
  Data Type Conversion81/1 -> Bus Creator/81  "RRR_FreespaceSectorKinestate77"
  Data Type Conversion82/1 -> Bus Creator/82  "RRR_FreespaceSectorKinestate78"
  Data Type Conversion83/1 -> Bus Creator/83  "RRR_FreespaceSectorKinestate79"
  Data Type Conversion84/1 -> Bus Creator/84  "RRR_FreespaceSectorKinestate80"
  Data Type Conversion85/1 -> Bus Creator/85  "RRR_FreespaceSectorKinestate81"
  Data Type Conversion86/1 -> Bus Creator/86  "RRR_FreespaceSectorKinestate82"
  Data Type Conversion87/1 -> Bus Creator/87  "RRR_FreespaceSectorKinestate83"
  Data Type Conversion88/1 -> Bus Creator/88  "RRR_FreespaceSectorKinestate84"
  Data Type Conversion89/1 -> Bus Creator/89  "RRR_FreespaceSectorKinestate85"
  Data Type Conversion90/1 -> Bus Creator/90  "RRR_FreespaceSectorKinestate86"
  Data Type Conversion91/1 -> Bus Creator/91  "RRR_FreespaceSectorKinestate87"
  Data Type Conversion92/1 -> Bus Creator/92  "RRR_FreespaceSectorKinestate88"
  Data Type Conversion93/1 -> Bus Creator/93  "RRR_FreespaceSectorKinestate89"
  Data Type Conversion94/1 -> Bus Creator/94  "RRR_FreespaceSectorKinestate90"
  Data Type Conversion95/1 -> Bus Creator/95  "RRR_FreespaceSectorKinestate91"
  Data Type Conversion96/1 -> Bus Creator/96  "RRR_FreespaceSectorKinestate92"
  Data Type Conversion97/1 -> Bus Creator/97  "RRR_FreespaceSectorKinestate93"
  Data Type Conversion98/1 -> Bus Creator/98  "RRR_FreespaceSectorKinestate94"
  Data Type Conversion99/1 -> Bus Creator/99  "RRR_FreespaceSectorKinestate95"
  Data Type Conversion100/1 -> Bus Creator/100  "RRR_FreespaceSectorKinestate96"
  Data Type Conversion101/1 -> Bus Creator/101  "RRR_FreespaceSectorKinestate97"
  Data Type Conversion102/1 -> Bus Creator/102  "RRR_FreespaceSectorKinestate98"
  Data Type Conversion103/1 -> Bus Creator/103  "RRR_FreespaceSectorKinestate99"
  Data Type Conversion104/1 -> Bus Creator/104  "RRR_RollingCounter_FSP_MSG3"
  Bus Creator/1 -> SRR_ADCU_RRR_Freespace_0x1EDFromOutData/1  "SRR_ADCU_RRR_Freespace_0x1EDFromOutData"
  SRR_ADCU_RRR_Freespace_0x1EDFromInData/1 -> CAN FD Unpack/1  "SRR_ADCU_RRR_Freespace_0x1EDFromInData"
